simulink model "encoder"  (R2023b)
settings: Solver=FixedStepDiscrete  StartTime=0.0  StopTime=10.0  FixedStep=0.01  RelTol=1e-3
values from neighbouring files (symbols this model uses):
  ANTI_CLOCKWISE_ROTATION = 2    [encoder_DD.sldd]
  CLOCKWISE_ROTATION = 1    [encoder_DD.sldd]
  ROTATION_DIRECTION_E : value not decoded    [encoder_DD.sldd]
libraries: simulink x7
settings Model: DataDictionary=encoder_DD.sldd  Creator=LENOVO-MCC  LastModifiedBy=LENOVO-MCC
settings OptimizationCC: DefaultParameterBehavior=Inlined  EnhancedBackFolding=on  PassReuseOutputArgsAs=Individual arguments  ZeroExternalMemoryAtStartup=off  ZeroInternalMemoryAtStartup=off  OptimizeBlockOrder=speed  DifferentSizesBufferReuse=on  OptimizationCustomize=off  EfficientTunableParamExpr=on
settings DebuggingCC: ParameterOverflowMsg=none  ParameterTunabilityLossMsg=error
settings SFSimCC: MATLABDynamicMemAlloc=off
settings RTWCC: Description=Embedded Coder  SystemTargetFile=ert.tlc  GenCodeOnly=on  TemplateMakefile=ert_default_tmf  GenerateReport=on  LaunchReport=on  GenerateCodeMetricsReport=on
settings CodeAppCC: ForceParamTrailComments=on  IgnoreCustomStorageClasses=off  OperatorAnnotations=on  SimulinkDataObjDesc=on  SFDataObjDesc=on  InsertBlockDesc=on
settings ERTTargetCC: TargetLangStandard=C99 (ISO)  GenerateSampleERTMain=on  InlinedParameterPlacement=NonHierarchical  ERTCustomFileTemplate=example_file_process.tlc

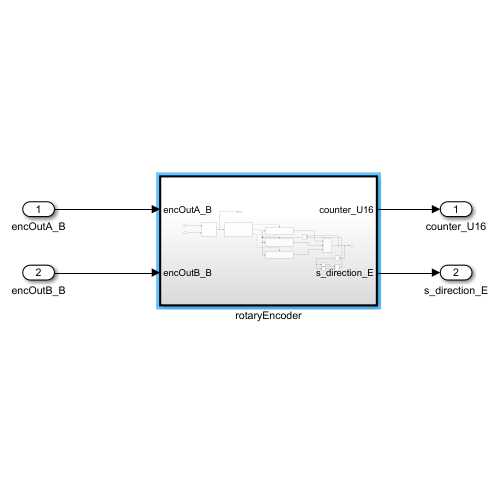
[thumbnail: Simulink's stored preview of the top-level diagram]
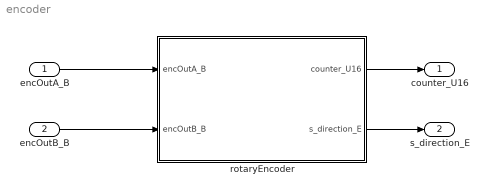
== system encoder ==
  encOutA_B : Inport  OutDataTypeStr=boolean
  encOutB_B : Inport  Port=2  OutDataTypeStr=boolean
  rotaryEncoder : Subsystem  TreatAsAtomicUnit=on
      settings: RTWFcnNameOpts=Use subsystem name  RTWFileNameOpts=Use subsystem name
  counter_U16 : Outport  OutDataTypeStr=uint16
  s_direction_E : Outport  Port=2  OutDataTypeStr=Enum: ROTATION_DIRECTION_E
  wires:
  encOutB_B/1 -> rotaryEncoder/2(encOutB_B)
  encOutA_B/1 -> rotaryEncoder/1(encOutA_B)
  rotaryEncoder/2(s_direction_E) -> s_direction_E/1
  rotaryEncoder/1(counter_U16) -> counter_U16/1

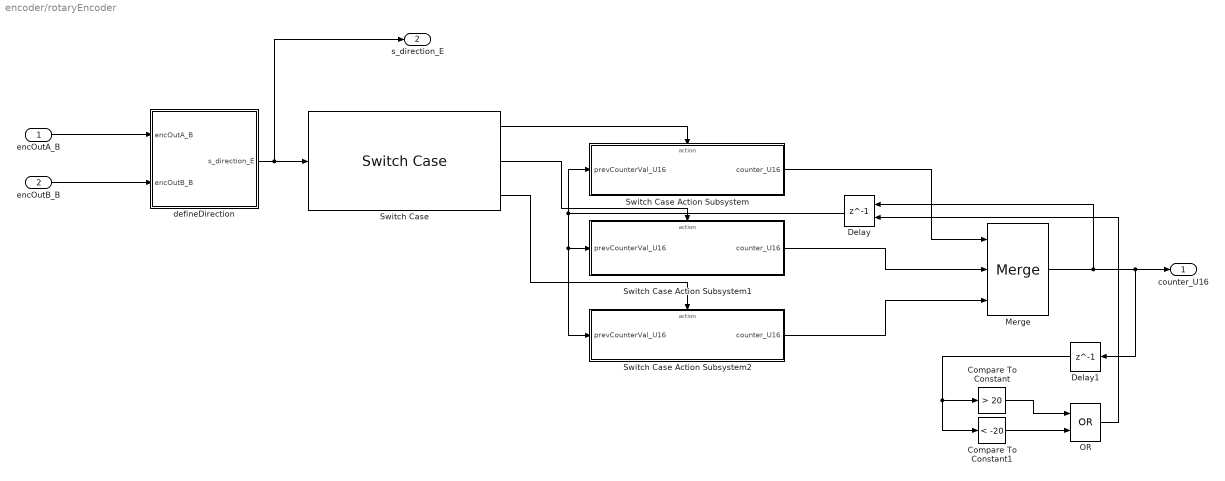
== system encoder/rotaryEncoder ==
  encOutA_B : Inport  OutDataTypeStr=boolean
  encOutB_B : Inport  Port=2  OutDataTypeStr=boolean
  Compare To Constant : simulink/Logic and Bit Operations/Compare To Constant  relop=>  const=20  OutDataTypeStr=boolean
  Compare To Constant1 : simulink/Logic and Bit Operations/Compare To Constant  relop=<  const=-20  OutDataTypeStr=boolean
  Delay : Delay  DelayLength=1  ExternalReset=Rising
      settings: InputPortMap=u0,r5
  Delay1 : Delay  DelayLength=1
  Merge : Merge  Inputs=3
  OR : Logic  Operator=OR  AllPortsSameDT=off  OutDataTypeStr=boolean
  Switch Case : SwitchCase  CaseConditions={ROTATION_DIRECTION_E.CLOCKWISE_ROTATION,ROTATION_DIRECTION_E.ANTI_CLOCKWISE_ROTATION}
  Switch Case Action Subsystem : Subsystem  TreatAsAtomicUnit=on
  Switch Case Action Subsystem1 : Subsystem  TreatAsAtomicUnit=on
  Switch Case Action Subsystem2 : Subsystem  TreatAsAtomicUnit=on
  defineDirection : Subsystem
  counter_U16 : Outport  OutDataTypeStr=uint16
  s_direction_E : Outport  Port=2  OutDataTypeStr=Enum: ROTATION_DIRECTION_E
  wires:
  encOutA_B/1 -> defineDirection/1(encOutA_B)
  encOutB_B/1 -> defineDirection/2(encOutB_B)
  defineDirection/1(s_direction_E) -> s_direction_E/1, Switch Case/1
  Switch Case/1 -> Switch Case Action Subsystem/Action
  Switch Case/2 -> Switch Case Action Subsystem1/Action
  Switch Case/3 -> Switch Case Action Subsystem2/Action
  Delay/1 -> Switch Case Action Subsystem/1(prevCounterVal_U16), Switch Case Action Subsystem2/1(prevCounterVal_U16), Switch Case Action Subsystem1/1(prevCounterVal_U16)
  Switch Case Action Subsystem/1(counter_U16) -> Merge/1
  Switch Case Action Subsystem1/1(counter_U16) -> Merge/2
  Switch Case Action Subsystem2/1(counter_U16) -> Merge/3
  Merge/1 -> Delay/1, Delay1/1, counter_U16/1
  Compare To Constant1/1 -> OR/2
  Compare To Constant/1 -> OR/1
  Delay1/1 -> Compare To Constant/1, Compare To Constant1/1
  OR/1 -> Delay/2

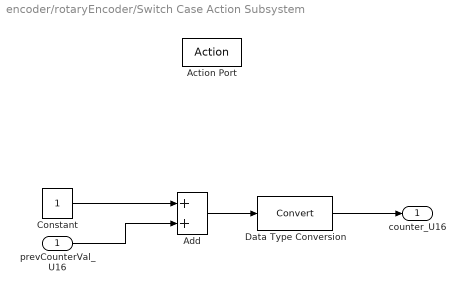
== system encoder/rotaryEncoder/Switch Case Action Subsystem ==
  prevCounterVal_U16 : Inport  OutDataTypeStr=uint16
  Action Port : ActionPort  ActionPortLabel=case [ CLOCKWISE_ROTATION ]:
  Add : Sum
  Constant : Constant  OutDataTypeStr=int8
  Data Type Conversion : DataTypeConversion  SaturateOnIntegerOverflow=off  RndMeth=Floor
  counter_U16 : Outport  OutDataTypeStr=uint16
  wires:
  Constant/1 -> Add/1
  prevCounterVal_U16/1 -> Add/2
  Add/1 -> Data Type Conversion/1
  Data Type Conversion/1 -> counter_U16/1

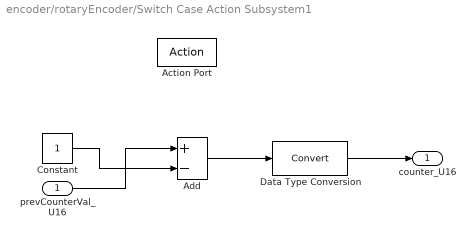
== system encoder/rotaryEncoder/Switch Case Action Subsystem1 ==
  prevCounterVal_U16 : Inport  OutDataTypeStr=uint16
  Action Port : ActionPort  ActionPortLabel=case [ ANTI_CLOCKWISE_ROTATION ]:
  Add : Sum  Inputs=+-
  Constant : Constant  OutDataTypeStr=int8
  Data Type Conversion : DataTypeConversion  SaturateOnIntegerOverflow=off  RndMeth=Floor
  counter_U16 : Outport  OutDataTypeStr=uint16
  wires:
  Add/1 -> Data Type Conversion/1
  prevCounterVal_U16/1 -> Add/1
  Constant/1 -> Add/2
  Data Type Conversion/1 -> counter_U16/1

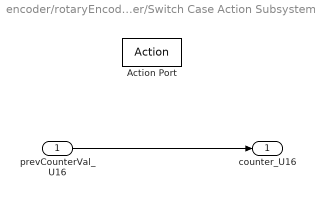
== system encoder/rotaryEncoder/Switch Case Action Subsystem2 ==
  prevCounterVal_U16 : Inport  OutDataTypeStr=uint16
  Action Port : ActionPort  ActionPortLabel=default:
  counter_U16 : Outport  OutDataTypeStr=uint16
  wires:
  prevCounterVal_U16/1 -> counter_U16/1

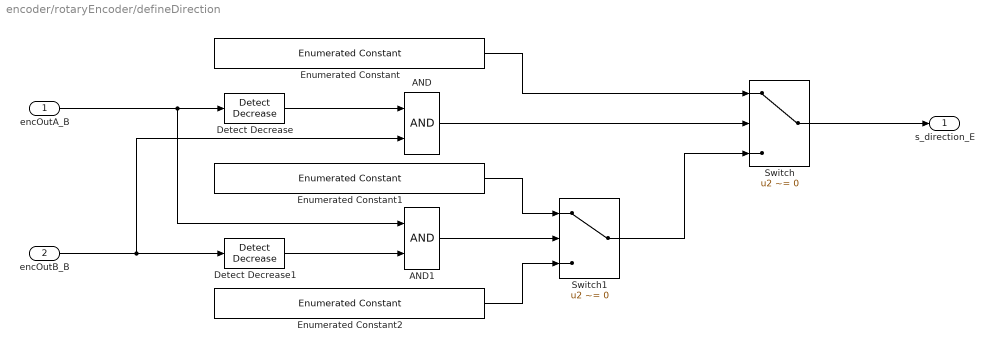
== system encoder/rotaryEncoder/defineDirection ==
  encOutA_B : Inport  OutDataTypeStr=boolean
  encOutB_B : Inport  Port=2  OutDataTypeStr=boolean
  AND : Logic  AllPortsSameDT=off  OutDataTypeStr=boolean
  AND1 : Logic  AllPortsSameDT=off  OutDataTypeStr=boolean
  Detect Decrease : simulink/Logic and Bit Operations/Detect Decrease  vinit=0.0  OutDataTypeStr=boolean
  Detect Decrease1 : simulink/Logic and Bit Operations/Detect Decrease  vinit=0.0  OutDataTypeStr=boolean
  Enumerated Constant : simulink/Sources/Enumerated Constant  OutDataTypeStr=Enum: ROTATION_DIRECTION_E  Value=ROTATION_DIRECTION_E.CLOCKWISE_ROTATION  SampleTime=inf
  Enumerated Constant1 : simulink/Sources/Enumerated Constant  OutDataTypeStr=Enum: ROTATION_DIRECTION_E  Value=ROTATION_DIRECTION_E.ANTI_CLOCKWISE_ROTATION  SampleTime=inf
  Enumerated Constant2 : simulink/Sources/Enumerated Constant  OutDataTypeStr=Enum: ROTATION_DIRECTION_E  Value=ROTATION_DIRECTION_E.NO_ROTATION  SampleTime=inf
  Switch : Switch  Criteria=u2 ~= 0  SaturateOnIntegerOverflow=off  InputSameDT=off
  Switch1 : Switch  Criteria=u2 ~= 0  SaturateOnIntegerOverflow=off  InputSameDT=off
  s_direction_E : Outport  OutDataTypeStr=Enum: ROTATION_DIRECTION_E
  wires:
  encOutB_B/1 -> AND/2, Detect Decrease1/1
  encOutA_B/1 -> AND1/1, Detect Decrease/1
  Detect Decrease/1 -> AND/1
  Detect Decrease1/1 -> AND1/2
  AND/1 -> Switch/2
  AND1/1 -> Switch1/2
  Enumerated Constant/1 -> Switch/1
  Enumerated Constant1/1 -> Switch1/1
  Enumerated Constant2/1 -> Switch1/3
  Switch1/1 -> Switch/3
  Switch/1 -> s_direction_E/1
